simulink model "SD_R3GDL"  (R2021b)
settings: Solver=VariableStepAuto  StartTime=0.0  StopTime=2  RelTol=1e-3
settings Model: Creator=alvar  LastModifiedBy=alvar

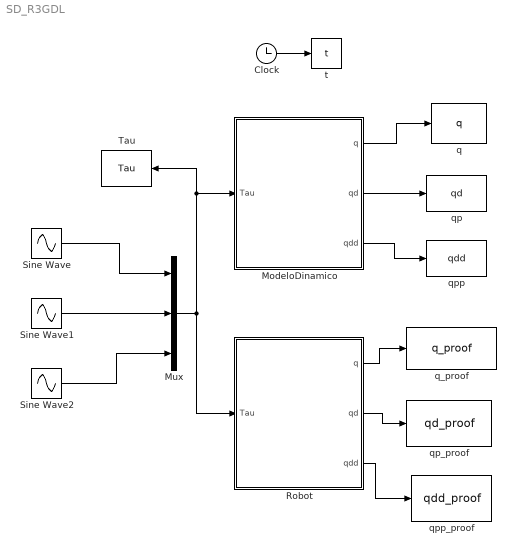
== system SD_R3GDL ==
  Clock : Clock
  ModeloDinamico : Subsystem
  Mux : Mux  Inputs=3
  Robot : Subsystem
      mask Display: image('C:\Users\alvar\OneDrive\Escritorio\TRABAJO CURSO\A_Análisis_Cinemático\3\robot3gdl.jpg'); % Use "Edit Image" on toolstrip to change.
  Sine Wave : Sin  Amplitude=10  SampleTime=0
  Sine Wave1 : Sin  Amplitude=10  Frequency=10  SampleTime=0
  Sine Wave2 : Sin  Amplitude=10  Frequency=5  SampleTime=0
  Tau : ToWorkspace  VariableName=Tau  SampleTime=-1
  q : ToWorkspace  VariableName=q  SampleTime=-1
  q_proof : ToWorkspace  VariableName=q_proof  SampleTime=-1
  qp : ToWorkspace  VariableName=qd  SampleTime=-1
  qp_proof : ToWorkspace  VariableName=qd_proof  SampleTime=-1
  qpp : ToWorkspace  VariableName=qdd  SampleTime=-1
  qpp_proof : ToWorkspace  VariableName=qdd_proof  SampleTime=-1
  t : ToWorkspace  VariableName=t  SampleTime=-1
  wires:
  Mux/1 -> Robot/1(Tau), Tau/1, ModeloDinamico/1(Tau)
  Sine Wave2/1 -> Mux/3
  Robot/1(q) -> q_proof/1
  Sine Wave/1 -> Mux/1
  Robot/3(qdd) -> qpp_proof/1
  Robot/2(qd) -> qp_proof/1
  ModeloDinamico/3(qdd) -> qpp/1
  Clock/1 -> t/1
  Sine Wave1/1 -> Mux/2
  ModeloDinamico/2(qd) -> qp/1
  ModeloDinamico/1(q) -> q/1

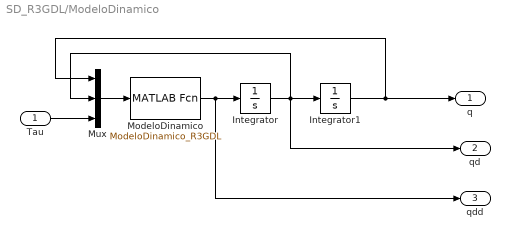
== system SD_R3GDL/ModeloDinamico ==
  Tau : Inport
  Integrator : Integrator  InitialCondition=[0;0;0];
  Integrator1 : Integrator  InitialCondition=[0 0 0]
  ModeloDinamico : MATLABFcn  MATLABFcn=ModeloDinamico_R3GDL  OutputDimensions=3
  Mux : Mux  Inputs=3
  q : Outport
  qd : Outport  Port=2
  qdd : Outport  Port=3
  wires:
  Mux/1 -> ModeloDinamico/1
  ModeloDinamico/1 -> Integrator/1, qdd/1
  Integrator/1 -> Integrator1/1, qd/1, Mux/2
  Integrator1/1 -> q/1, Mux/1
  Tau/1 -> Mux/3

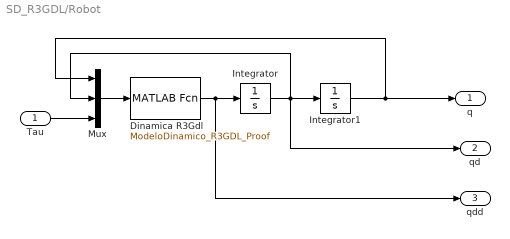
== system SD_R3GDL/Robot ==
  Tau : Inport
  Dinamica R3Gdl : MATLABFcn  MATLABFcn=ModeloDinamico_R3GDL_Proof  OutputDimensions=3
  Integrator : Integrator  InitialCondition=[0;0;0];
  Integrator1 : Integrator  InitialCondition=[0 0 0]
  Mux : Mux  Inputs=3
  q : Outport
  qd : Outport  Port=2
  qdd : Outport  Port=3
  wires:
  Mux/1 -> Dinamica R3Gdl/1
  Dinamica R3Gdl/1 -> Integrator/1, qdd/1
  Integrator/1 -> Integrator1/1, qd/1, Mux/2
  Integrator1/1 -> q/1, Mux/1
  Tau/1 -> Mux/3
